simulink model "SMA_scamless"  (R2022a)
settings: Solver=VariableStepAuto  StartTime=0.0  StopTime=0.1  RelTol=1e-3
InitFcn:
  | g = 9.8;
  | l = 0.05; % m
  | L = 0.3;
  | m = 40; % mass to be lifted
  | 
  | % spring parameters
  | E = 40000; % approx. (gets cancelled in calculations)
  | G = E/2/(1+0.33);
  | D = 0.025; % spring dia
  | d = 0.005; % wire dia
  | l_sp = 0.10; % length of spring actuator
  | C = 5; % spring index
  | Kw = (4*C-1)/(4*C-4) + 0.615/C;
  | K_TF = 8*D*Kw/(pi*d^3); % gain between shear stress and force
  | na = 52; % number of active coils
  | k_sp = 24*G*d^4/(8*D^3*na); % combined spring constant
  | K_TE = E/(K_TF*k_sp*l); % gain between theta and epsilon
  | K_xE = E/(K_TF*k_sp); % between displacment and epsilon
undefined symbols (not defined in the file): Af, As, cA, cM, eps_L, Mf, Ms, xi0, Ya, Ym
settings Model: SnapshotInterval=1  Creator=ashut  LastModifiedBy=ashut

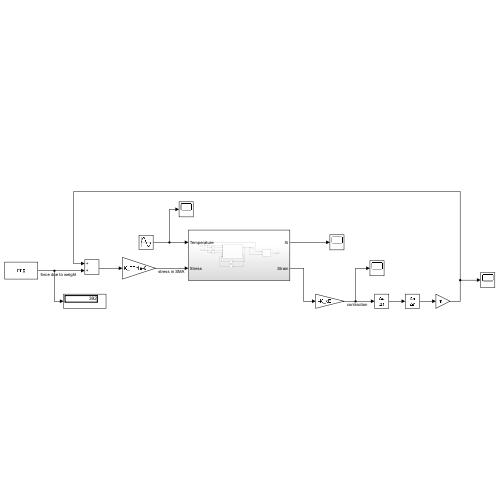
[thumbnail: Simulink's stored preview of the top-level diagram]
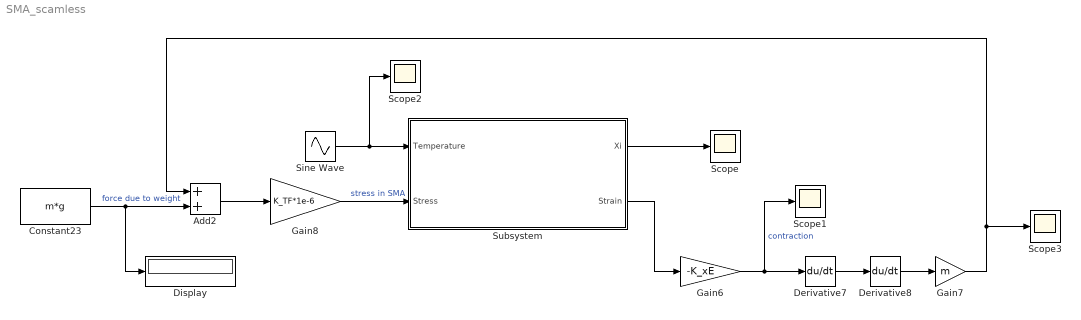
== system SMA_scamless ==
  Add2 : Sum
  Constant23 : Constant  Value=m*g
  Derivative7 : Derivative
  Derivative8 : Derivative
  Display : Display
  Gain6 : Gain  Gain=-K_xE
  Gain7 : Gain  Gain=m
  Gain8 : Gain  Gain=K_TF*1e-6
  Scope{,1..3} (4 alike) : Scope
  Sine Wave : Sin  Amplitude=40  Bias=60  Frequency=20  SampleTime=0
  Subsystem : Subsystem  InitFcn=|
      | xi0 = 0.5; % initial xi value
      | 
      | Mf = 9;
      | Ms = 18;
      | As = 35;
      | Af = 49;
      | cM = 8;
      | cA = 13;
      | 
      | Ya = 67000; % MPa
      | Ym = 24000;
      | eps_L = 0.07; % max recoverable strain
  wires:
  Subsystem/1(Xi) -> Scope/1
  Subsystem/2(Strain) -> Gain6/1
  Sine Wave/1 -> Scope2/1, Subsystem/1(Temperature)
  Derivative8/1 -> Gain7/1
  Gain6/1 -> Scope1/1, Derivative7/1  "contraction"
  Derivative7/1 -> Derivative8/1
  Gain7/1 -> Scope3/1, Add2/1
  Constant23/1 -> Display/1, Add2/2  "force due to weight"
  Add2/1 -> Gain8/1
  Gain8/1 -> Subsystem/2(Stress)  "stress in SMA"

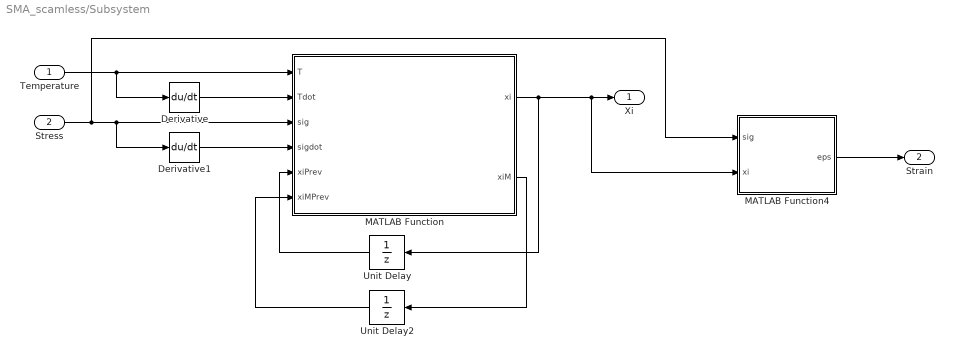
== system SMA_scamless/Subsystem ==
  Temperature : Inport
  Stress : Inport  Port=2
  Derivative : Derivative
  Derivative1 : Derivative
  MATLAB Function : MATLAB Function  TreatAsAtomicUnit=on
  MATLAB Function4 : MATLAB Function  TreatAsAtomicUnit=on
  Unit Delay : UnitDelay  InitialCondition=xi0  SampleTime=-1  HasFrameUpgradeWarning=on
  Unit Delay2 : UnitDelay  InitialCondition=xi0  SampleTime=-1  HasFrameUpgradeWarning=on
  Xi : Outport
  Strain : Outport  Port=2
  wires:
  Temperature/1 -> Derivative/1, MATLAB Function/1(T)
  MATLAB Function/2(xiM) -> Unit Delay2/1
  Derivative/1 -> MATLAB Function/2(Tdot)
  Unit Delay/1 -> MATLAB Function/5(xiPrev)
  Derivative1/1 -> MATLAB Function/4(sigdot)
  Unit Delay2/1 -> MATLAB Function/6(xiMPrev)
  MATLAB Function/1(xi) -> MATLAB Function4/2(xi), Xi/1, Unit Delay/1
  Stress/1 -> MATLAB Function4/1(sig), Derivative1/1, MATLAB Function/3(sig)
  MATLAB Function4/1(eps) -> Strain/1

== matlab function SMA_scamless/Subsystem/MATLAB Function ==
  data: T input; xi output; Tdot input; sig input; sigdot input; xiPrev input; xiM output; xiMPrev input; Ms parameter; Mf parameter; As parameter; Af parameter; cM parameter; cA parameter
function [xi, xiM]= fcn(T, Tdot, sig, sigdot, xiPrev, xiMPrev, Ms, Mf, As, Af, cM, cA)
    
    % hold by default (if any changes are to be made, they're made in if
    % else blocks below)
    % this is what happens in the middle region (out of mart or aust)
    xi = xiPrev;
    xiM = xiMPrev;

    Mf_mod = Mf + sig/cM;
    Ms_mod = Ms + sig/cM;
    As_mod = As + sig/cA;
    Af_mod = Af + sig/cA;

    if T > Mf_mod && T < Ms_mod
        cosTerm = cos(pi/(Ms-Mf)*(T-Mf-sig/cM)); % cos term in martensite region

        if Tdot > sigdot/cM
            if cosTerm == 1 % to prevent division by zero
                xiM = 1;
            else
                xiM = (2*xi - 1 - cosTerm)/(1 - cosTerm);
            end
        elseif Tdot < sigdot/cM
            xi = (1+xiM)/2 + (1-xiM)/2*cosTerm;
        end

    elseif T > As_mod && T < Af_mod
        cosTerm = cos(pi/(Af-As)*(T-As-sig/cA)); % cos term in austenite region

        if Tdot < sigdot/cA
            if cosTerm == -1 % to prevent divison by zero
                xiM = 1;
            else
                xiM = 2*xi/(1+cosTerm);
            end
        elseif Tdot > sigdot/cA
            xi = xiM/2*(1+cosTerm);
        end

    elseif T <= Mf_mod
        xi = 1;
        xiM = 1;
    elseif T >= Af_mod
        xi = 0;
        xiM = 0;
    end

== matlab function SMA_scamless/Subsystem/MATLAB Function4 ==
  data: sig input; xi input; eps output; Ya parameter; Ym parameter; eps_L parameter; xi0 parameter
function eps = fcn(sig, xi, Ya, Ym, eps_L, xi0)

Y = Ya + (Ym-Ya)*xi;
Y0 = Ya + (Ym-Ya)*xi0;
eps = (sig + eps_L*(Y*xi - Y0*xi0))/Y;
